simulink model "TestFlow"  (R2013b)
settings: Solver=ode45  StartTime=0.0  StopTime=10.0  RelTol=1e-3
settings Model: Creator=qiji  LastModifiedBy=qiji

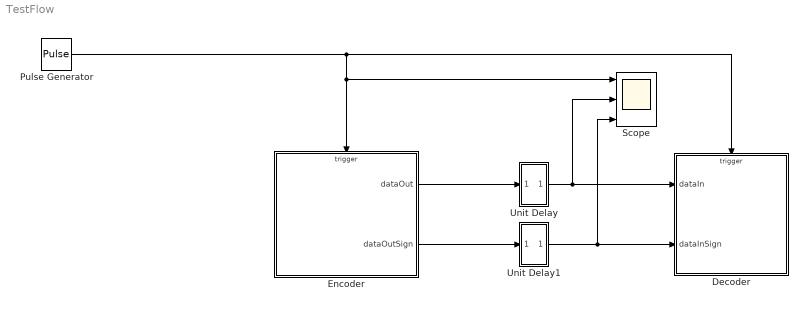
== system TestFlow ==
  Decoder : Stateflow chart  TreatAsAtomicUnit=on
  Encoder : Stateflow chart  TreatAsAtomicUnit=on
  Pulse Generator : DiscretePulseGenerator  PulseType=Time based  Period=0.1  PulseWidth=50
  Scope : Scope  NumInputPorts=3
      settings: TimeRange=10  YMin=0.95~-1~-5  YMax=1.05~1~5
  Unit Delay : Subsystem
  Unit Delay1 : Subsystem
  wires:
  Pulse Generator/1 -> Decoder/Trigger, Encoder/Trigger, Scope/1
  Encoder/1(dataOut) -> Unit Delay/1(In1)
  Encoder/2(dataOutSign) -> Unit Delay1/1(In1)
  Unit Delay/1(Out1) -> Scope/2, Decoder/1(dataIn)
  Unit Delay1/1(Out1) -> Scope/3, Decoder/2(dataInSign)

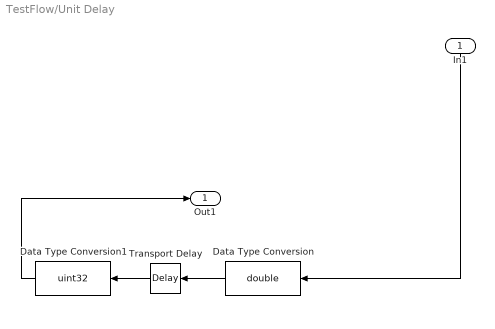
== system TestFlow/Unit Delay ==
  In1 : Inport
  Data Type Conversion : DataTypeConversion  OutDataTypeStr=double
  Data Type Conversion1 : DataTypeConversion  OutDataTypeStr=uint32
  Transport Delay : TransportDelay  DelayTime=1e-7
  Out1 : Outport
  wires:
  In1/1 -> Data Type Conversion/1
  Data Type Conversion/1 -> Transport Delay/1
  Transport Delay/1 -> Data Type Conversion1/1
  Data Type Conversion1/1 -> Out1/1

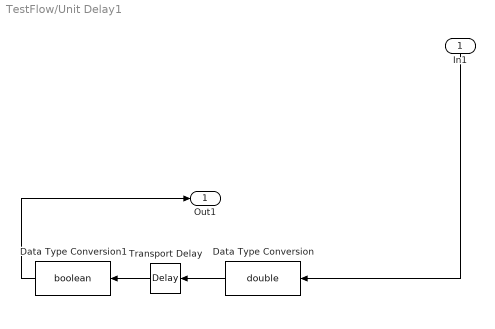
== system TestFlow/Unit Delay1 ==
  In1 : Inport
  Data Type Conversion : DataTypeConversion  OutDataTypeStr=double
  Data Type Conversion1 : DataTypeConversion  OutDataTypeStr=boolean
  Transport Delay : TransportDelay  DelayTime=1e-7
  Out1 : Outport
  wires:
  In1/1 -> Data Type Conversion/1
  Data Type Conversion/1 -> Transport Delay/1
  Transport Delay/1 -> Data Type Conversion1/1
  Data Type Conversion1/1 -> Out1/1

== stateflow chart TestFlow/Encoder ==
  state Encoding [parallel]
    settings: executionOrder=1
    state trans
      entry:
      count = 0;
      trans -> trans [order 1] : CLK
          | {
          | dataOut = bitoperate.getbit(input);
          | input = bitoperate.shiftbit(input, 1);
          | count++;
          | }
    state start
    (default) -> start : {
        | init()
        | }
    trans -> start [order 1] : [count == 32]
        | {
        | dataOut = 0;
        | bufferIndex++;
        | dataOutSign = false;
        | }
    start -> trans [order 2] : CLK
        | {
        | input = bitoperate.ManchesterEncoding(buffer[bufferIndex]);
        | dataOutSign = true;
        | }
    start -> Encoding [order 1] : [bufferIndex==bufferSize+1]
  state init [function]
    (default) -> (junction 65) : {
        | buffer[1]=36864;
        | buffer[2]=32768;
        | bufferSize=2;
        | bufferIndex=1;
        | }
  state bitoperate [group]
  data: num function_input uint32; r function_output uint32; data function_input uint32; num function_input uint32; r function_output uint32; data function_input uint32; r function_output uint32; dataOut output uint32; input local uint32; count local double; buffer local uint32 size=100; bufferSize local double; bufferIndex local double; dataOutSign output boolean
  events: CLK input EITHER_EDGE_EVENT
  function r = getbit(num):
    | function r = getbit(num)
    | r = bitget(num, 32);
  function r = shiftbit(data, num):
    | function r = shiftbit(data, num)
    | r = bitshift(data, num);
    | %for i=1:cnt
    | %   r = bitset(r, i, 0);
    | %end
  function r = ManchesterEncoding(data):
    | function r = ManchesterEncoding(data)
    | r = data;
    | for i = 1:16
    |     x = bitget(data, i);
    |     if x == 0
    |         r = bitset(r, i*2-1, 1);
    |         r = bitset(r, i*2, 0);
    |     else
    |         r = bitset(r, i*2-1, 0);
    |         r = bitset(r, i*2, 1);
    |     end
    | end

== stateflow chart TestFlow/Decoder ==
  state bitoperate [group]
  state start
  state decode
    decode -> decode [order 1] : CLK
        | {
        | ans = bitoperate.shiftbit(ans, 1) + dataIn;
        | count++;
        | }
  start -> decode : [dataInSign==true]
      | {
      | ans = 0;
      | count = 0;
      | }
  (default) -> start
  decode -> start [order 1] : [count==32]
      | {
      | ans = ManchesterDecoding(ans);
      | }
  data: num function_input uint32; r function_output uint32; data function_input uint32; num function_input uint32; r function_output uint32; r function_output uint32; data function_input uint32; dataIn input uint32; ans local uint32; dataInSign input boolean; count local uint32
  events: CLK input EITHER_EDGE_EVENT
  function r = getbit(num):
    | function r = getbit(num)
    | r = bitget(num, 32);
  function r = shiftbit(data, num):
    | function r = shiftbit(data, num)
    | r = bitshift(data, num);
    | %for i=1:cnt
    | %   r = bitset(r, i, 0);
    | %end
  function r = ManchesterDecoding(data):
    | function r = ManchesterDecoding(data)
    | r = uint32(0);
    | for i = (1:2:32)
    |     x0 = bitget(data, i);
    |     x1 = bitget(data, i+1);
    |     if x0==0 && x1==1
    |         r = bitset(r, (i+1)/2, 1);
    |     else
    |         r = bitset(r, (i+1)/2, 0);
    |     end
    | end
